simulink model "CAN_Model"  (R2018a)
settings: Solver=VariableStepAuto  StartTime=0.0  StopTime=12.4  RelTol=1e-3
InitFcn:
  | clc;
  | clear;
  | 
  | readyToSend = 1;
libraries: simulink_extras x2
settings Model: Creator=Emiliano  LastModifiedBy=Emiliano

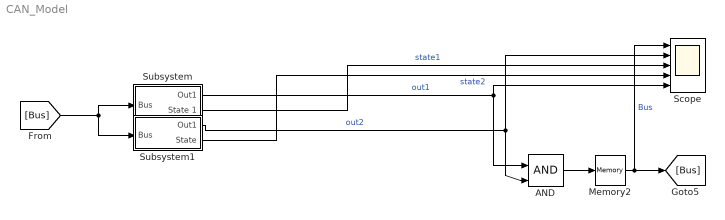
== system CAN_Model ==
  AND : Logic  IconShape=distinctive  AllPortsSameDT=off  OutDataTypeStr=boolean
  Memory2 : Memory  InitialCondition=1  InheritSampleTime=on
  Scope : Scope  NumInputPorts=5
  Subsystem : Subsystem
  Subsystem1 : Subsystem
  wires:
  AND/1 -> Memory2/1
  Memory2/1 -> Scope/1, [Bus]  "Bus"
  Subsystem/1(Out1) -> Scope/5, AND/1  "out1"
  Subsystem1/1(Out1) -> AND/2, Scope/2  "out2"
  [Bus] -> Subsystem1/1("Bus "), Subsystem/1("Bus ")
  Subsystem/2(State 1) -> Scope/3  "state1"
  Subsystem1/2("State ") -> Scope/4  "state2"

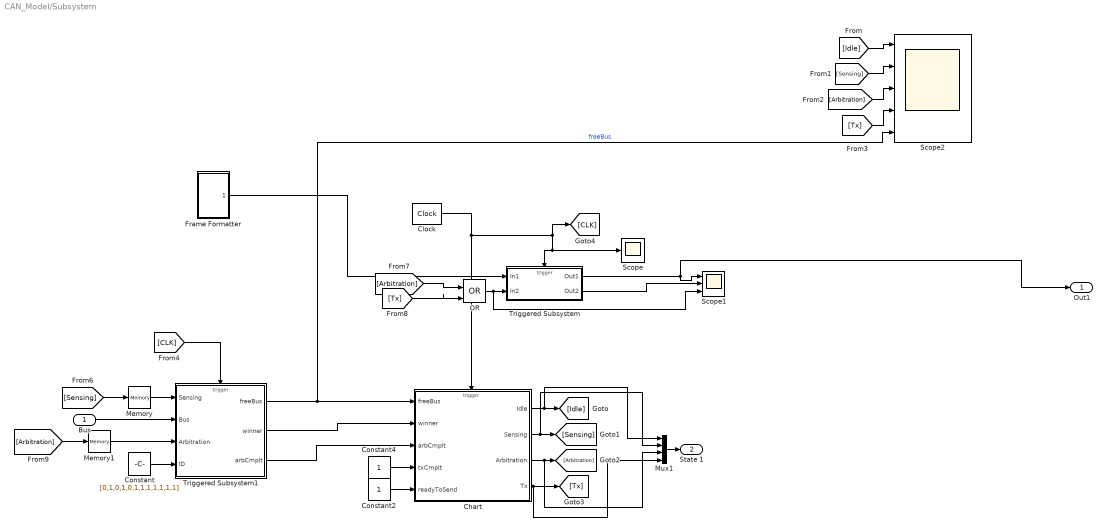
== system CAN_Model/Subsystem ==
  "Bus " : Inport
  Chart : Stateflow chart  TreatAsAtomicUnit=on
  Clock : simulink_extras/Flip Flops/Clock  period=0.2
  Constant : Constant  Value=[0,1,0,1,0,1,1,1,1,1,1,1]
  Constant2 : Constant
  Constant4 : Constant
  Frame Formatter : Subsystem
  Memory : Memory  InheritSampleTime=on
  Memory1 : Memory
  Mux1 : Mux
  OR : Logic  Operator=OR  IconShape=distinctive  AllPortsSameDT=off  OutDataTypeStr=boolean
  Scope : Scope
  Scope1 : Scope  NumInputPorts=3
  Scope2 : Scope  NumInputPorts=5
  Triggered Subsystem : Subsystem  TreatAsAtomicUnit=on
  Triggered Subsystem1 : Subsystem  TreatAsAtomicUnit=on
  Out1 : Outport
  State 1 : Outport  Port=2
  wires:
  Constant/1 -> Triggered Subsystem1/4(ID)
  Clock/1 -> Chart/Trigger, [CLK], Triggered Subsystem/Trigger, Scope/1
  OR/1 -> Scope1/3, Triggered Subsystem/2(In2)
  [Arbitration] -> OR/1
  Memory1/1 -> Triggered Subsystem1/3("Arbitration ")
  Triggered Subsystem1/3(arbCmplt) -> Chart/3(arbCmplt)
  Triggered Subsystem1/2(winner) -> Chart/2(winner)
  [Idle] -> Scope2/1
  [Tx] -> OR/2
  Constant2/1 -> Chart/5(readyToSend)
  [Arbitration] -> Memory1/1
  Memory/1 -> Triggered Subsystem1/1(Sensing)
  Triggered Subsystem1/1("freeBus ") -> Chart/1(freeBus), Scope2/5  "freeBus"
  [CLK] -> Triggered Subsystem1/Trigger
  [Sensing] -> Memory/1
  Frame Formatter/1(Frame) -> Triggered Subsystem/1(In1)
  Constant4/1 -> Chart/4(txCmplt)
  Triggered Subsystem/2(Out2) -> Scope1/2
  Triggered Subsystem/1(Out1) -> Out1/1, Scope1/1
  [Tx] -> Scope2/4
  [Arbitration] -> Scope2/3
  [Sensing] -> Scope2/2
  "Bus "/1 -> Triggered Subsystem1/2(Bus)
  Chart/2(" Sensing") -> [Sensing], Mux1/2
  Chart/4(" Tx") -> Mux1/4, [Tx]
  Chart/1(" Idle") -> [Idle], Mux1/1
  Chart/3(" Arbitration") -> Mux1/3, [Arbitration]
  Mux1/1 -> State 1/1

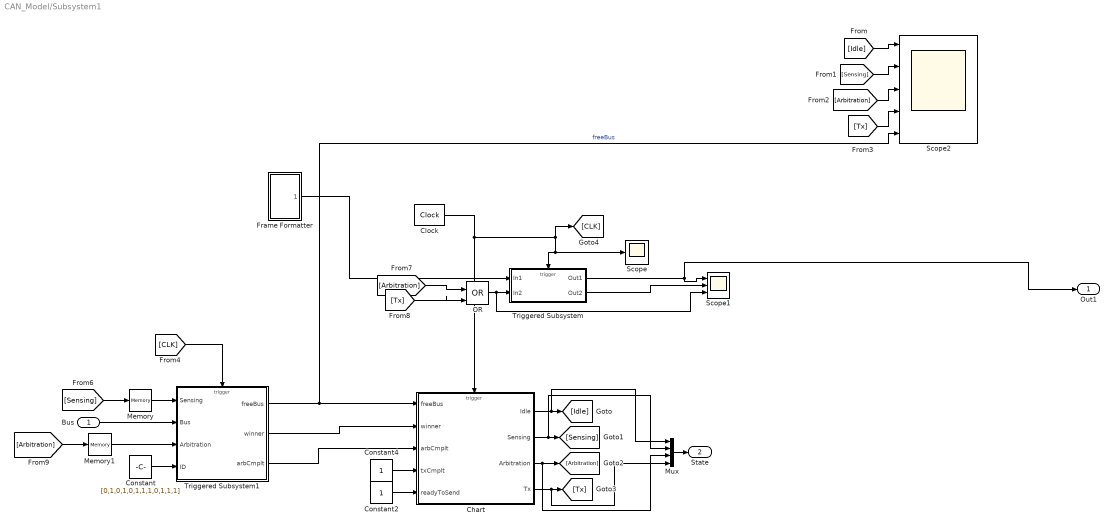
== system CAN_Model/Subsystem1 ==
  "Bus " : Inport
  Chart : Stateflow chart  TreatAsAtomicUnit=on
  Clock : simulink_extras/Flip Flops/Clock  period=0.2
  Constant : Constant  Value=[0,1,0,1,0,1,1,1,0,1,1,1]
  Constant2 : Constant
  Constant4 : Constant
  Frame Formatter : Subsystem
  Memory : Memory  InheritSampleTime=on
  Memory1 : Memory
  Mux : Mux
  OR : Logic  Operator=OR  IconShape=distinctive  AllPortsSameDT=off  OutDataTypeStr=boolean
  Scope : Scope
  Scope1 : Scope  NumInputPorts=3
  Scope2 : Scope  NumInputPorts=5
  Triggered Subsystem : Subsystem  TreatAsAtomicUnit=on
  Triggered Subsystem1 : Subsystem  TreatAsAtomicUnit=on
  Out1 : Outport
  "State " : Outport  Port=2
  wires:
  Constant/1 -> Triggered Subsystem1/4(ID)
  Clock/1 -> Chart/Trigger, [CLK], Triggered Subsystem/Trigger, Scope/1
  OR/1 -> Scope1/3, Triggered Subsystem/2(In2)
  [Arbitration] -> OR/1
  Memory1/1 -> Triggered Subsystem1/3("Arbitration ")
  Triggered Subsystem1/3(arbCmplt) -> Chart/3(arbCmplt)
  Triggered Subsystem1/2(winner) -> Chart/2(winner)
  [Idle] -> Scope2/1
  [Tx] -> OR/2
  Constant2/1 -> Chart/5(readyToSend)
  [Arbitration] -> Memory1/1
  Memory/1 -> Triggered Subsystem1/1(Sensing)
  Chart/4(" Tx") -> Mux/4, [Tx]
  Triggered Subsystem1/1("freeBus ") -> Chart/1(freeBus), Scope2/5  "freeBus"
  Chart/2(" Sensing") -> Mux/2, [Sensing]
  [CLK] -> Triggered Subsystem1/Trigger
  Chart/1(" Idle") -> Mux/1, [Idle]
  Chart/3(" Arbitration") -> Mux/3, [Arbitration]
  [Sensing] -> Memory/1
  Frame Formatter/1(Frame) -> Triggered Subsystem/1(In1)
  Constant4/1 -> Chart/4(txCmplt)
  Triggered Subsystem/2(Out2) -> Scope1/2
  Triggered Subsystem/1(Out1) -> Out1/1, Scope1/1
  [Tx] -> Scope2/4
  [Arbitration] -> Scope2/3
  [Sensing] -> Scope2/2
  "Bus "/1 -> Triggered Subsystem1/2(Bus)
  Mux/1 -> "State "/1

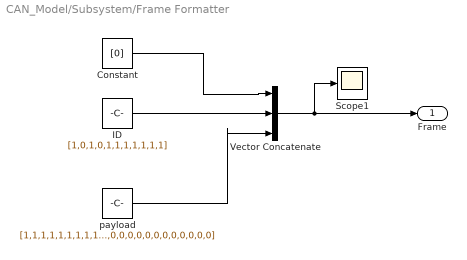
== system CAN_Model/Subsystem/Frame Formatter ==
  Constant : Constant  Value=[0]
  ID : Constant  Value=[1,0,1,0,1,1,1,1,1,1,1]
  Scope1 : Scope
  Vector Concatenate : Concatenate  NumInputs=3
  "payload " : Constant  Value=[1,1,1,1,1,1,1,1,1,1,1,1,1,1,1,1,1,1,1,1,1,1,1,1,1,0,0,0,0,0,0,0,0,0,0,0,0,0,0,0,0,0,0,0,0,0,0,0,0,0]
  Frame : Outport
  wires:
  ID/1 -> Vector Concatenate/2
  Constant/1 -> Vector Concatenate/1
  "payload "/1 -> Vector Concatenate/3
  Vector Concatenate/1 -> Frame/1, Scope1/1

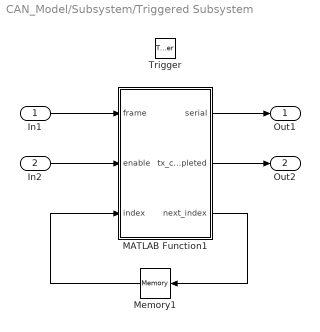
== system CAN_Model/Subsystem/Triggered Subsystem ==
  In1 : Inport
  In2 : Inport  Port=2
  Trigger : TriggerPort  VariantControl=Variant
  MATLAB Function1 : MATLAB Function  TreatAsAtomicUnit=on
  Memory1 : Memory  InitialCondition=1  InheritSampleTime=on
  Out1 : Outport
  Out2 : Outport  Port=2
  wires:
  In1/1 -> MATLAB Function1/1(frame)
  Memory1/1 -> MATLAB Function1/3(index)
  MATLAB Function1/1(serial) -> Out1/1
  MATLAB Function1/3(next_index) -> Memory1/1
  MATLAB Function1/2(tx_completed) -> Out2/1
  In2/1 -> MATLAB Function1/2(enable)

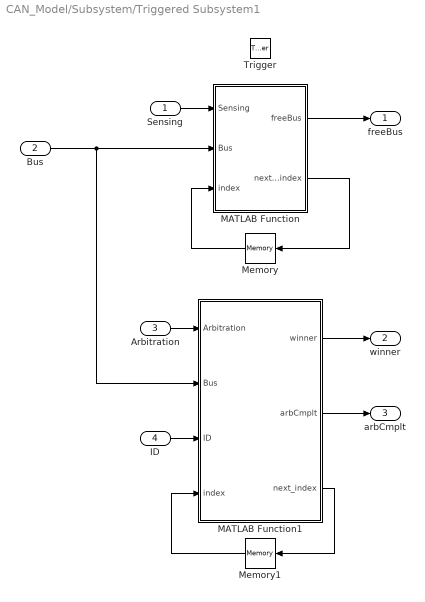
== system CAN_Model/Subsystem/Triggered Subsystem1 ==
  Sensing : Inport
  Bus : Inport  Port=2
  "Arbitration " : Inport  Port=3
  ID : Inport  Port=4
  Trigger : TriggerPort  VariantControl=Variant
  MATLAB Function : MATLAB Function  TreatAsAtomicUnit=on
  MATLAB Function1 : MATLAB Function  TreatAsAtomicUnit=on
  Memory : Memory  InheritSampleTime=on
  Memory1 : Memory  InitialCondition=1  InheritSampleTime=on
  "freeBus " : Outport
  winner : Outport  Port=2
  arbCmplt : Outport  Port=3
  wires:
  Sensing/1 -> MATLAB Function/1(Sensing)
  Bus/1 -> MATLAB Function1/2(Bus), MATLAB Function/2(Bus)
  MATLAB Function/2(next_index) -> Memory/1
  Memory/1 -> MATLAB Function/3(index)
  MATLAB Function/1(freeBus) -> "freeBus "/1
  "Arbitration "/1 -> MATLAB Function1/1(Arbitration)
  MATLAB Function1/3(next_index) -> Memory1/1
  Memory1/1 -> MATLAB Function1/4(index)
  ID/1 -> MATLAB Function1/3(ID)
  MATLAB Function1/2(arbCmplt) -> arbCmplt/1
  MATLAB Function1/1(winner) -> winner/1

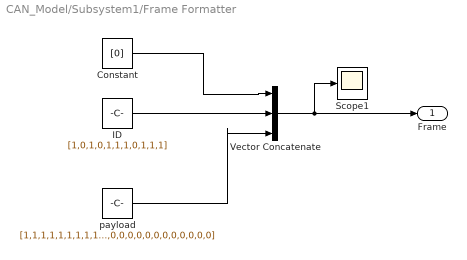
== system CAN_Model/Subsystem1/Frame Formatter ==
  Constant : Constant  Value=[0]
  ID : Constant  Value=[1,0,1,0,1,1,1,0,1,1,1]
  Scope1 : Scope
  Vector Concatenate : Concatenate  NumInputs=3
  "payload " : Constant  Value=[1,1,1,1,1,1,1,1,1,1,1,1,1,1,1,1,1,1,1,1,1,1,1,1,1,0,0,0,0,0,0,0,0,0,0,0,0,0,0,0,0,0,0,0,0,0,0,0,0,0]
  Frame : Outport
  wires:
  ID/1 -> Vector Concatenate/2
  Constant/1 -> Vector Concatenate/1
  "payload "/1 -> Vector Concatenate/3
  Vector Concatenate/1 -> Frame/1, Scope1/1

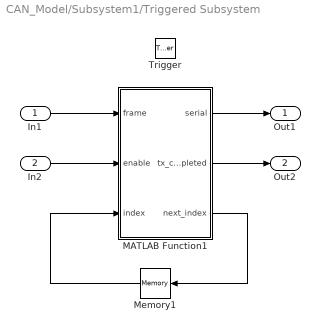
== system CAN_Model/Subsystem1/Triggered Subsystem ==
  In1 : Inport
  In2 : Inport  Port=2
  Trigger : TriggerPort  VariantControl=Variant
  MATLAB Function1 : MATLAB Function  TreatAsAtomicUnit=on
  Memory1 : Memory  InitialCondition=1  InheritSampleTime=on
  Out1 : Outport
  Out2 : Outport  Port=2
  wires:
  In1/1 -> MATLAB Function1/1(frame)
  Memory1/1 -> MATLAB Function1/3(index)
  MATLAB Function1/1(serial) -> Out1/1
  MATLAB Function1/3(next_index) -> Memory1/1
  MATLAB Function1/2(tx_completed) -> Out2/1
  In2/1 -> MATLAB Function1/2(enable)

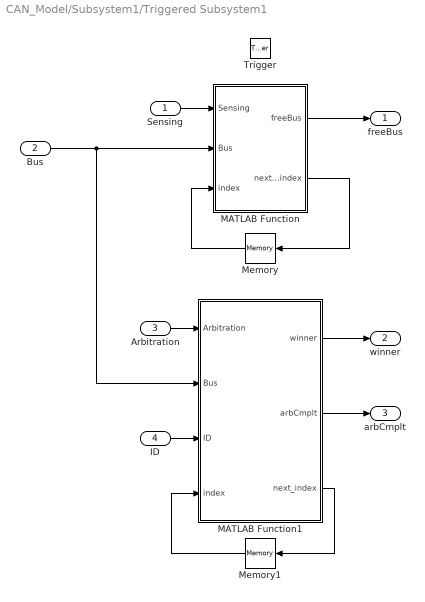
== system CAN_Model/Subsystem1/Triggered Subsystem1 ==
  Sensing : Inport
  Bus : Inport  Port=2
  "Arbitration " : Inport  Port=3
  ID : Inport  Port=4
  Trigger : TriggerPort  VariantControl=Variant
  MATLAB Function : MATLAB Function  TreatAsAtomicUnit=on
  MATLAB Function1 : MATLAB Function  TreatAsAtomicUnit=on
  Memory : Memory  InheritSampleTime=on
  Memory1 : Memory  InitialCondition=1  InheritSampleTime=on
  "freeBus " : Outport
  winner : Outport  Port=2
  arbCmplt : Outport  Port=3
  wires:
  Sensing/1 -> MATLAB Function/1(Sensing)
  Bus/1 -> MATLAB Function1/2(Bus), MATLAB Function/2(Bus)
  MATLAB Function/2(next_index) -> Memory/1
  Memory/1 -> MATLAB Function/3(index)
  MATLAB Function/1(freeBus) -> "freeBus "/1
  "Arbitration "/1 -> MATLAB Function1/1(Arbitration)
  MATLAB Function1/3(next_index) -> Memory1/1
  Memory1/1 -> MATLAB Function1/4(index)
  ID/1 -> MATLAB Function1/3(ID)
  MATLAB Function1/2(arbCmplt) -> arbCmplt/1
  MATLAB Function1/1(winner) -> winner/1

== matlab function CAN_Model/Subsystem/Triggered Subsystem1/MATLAB Function ==
  data: Sensing input; freeBus output; Bus input; index input; next_index output
function [freeBus, next_index] = fcn(Sensing, Bus, index)

freeBus = 0;

if Sensing == 1
    if Bus == 1
        if index < 10
            next_index = index + 1;
        else
            next_index = 0;
            freeBus = 1;
        end
    else
        next_index = 0;
    end
else
   next_index = 0;
end

end

== matlab function CAN_Model/Subsystem/Triggered Subsystem/MATLAB Function1 ==
  data: frame input; enable input; serial output; tx_completed output; index input; next_index output
function [serial,  tx_completed ,next_index]  = fcn(frame, enable, index)

if enable == 1
frame_size = size(frame);
if index > frame_size
    serial = 1;
    tx_completed = 1;
    next_index = 1;
else
    serial = frame(index);
    next_index = index + 1;
    tx_completed = 0;
end
else
    tx_completed = 0;
    serial = 1;
    next_index = 1;
end

end

== stateflow chart CAN_Model/Subsystem/Chart ==
  settings: executeAtInitialization=1
  state Idle
  state Sensing
  state Tx
  state Arbitration
  (default) -> Idle
  Idle -> Idle [order 2] : [readyToSend == 0]
  Idle -> Sensing [order 1] : [readyToSend > 0]
  Tx -> Idle [order 1] : [txCmplt == 1]
  Sensing -> Sensing [order 1] : [freeBus == 0]
  Arbitration -> Sensing [order 2] : [winner == 0 && arbCmplt == 1]
  Tx -> Tx [order 2] : [txCmplt == 0]
  Sensing -> Arbitration [order 2] : [freeBus == 1]
  Arbitration -> Tx [order 1] : [winner == 1 && arbCmplt == 1]
  Arbitration -> Arbitration [order 3] : [arbCmplt == 0]
  data: freeBus input; winner input; Idle output boolean; Sensing output boolean; Arbitration output boolean; Tx output boolean; arbCmplt input; txCmplt input; readyToSend input
  events: Start input RISING_EDGE_EVENT

== matlab function CAN_Model/Subsystem/Triggered Subsystem1/MATLAB Function1 ==
  data: winner output; arbCmplt output; Arbitration input; Bus input; ID input; next_index output; index input
function [winner, arbCmplt, next_index] = fcn(Arbitration, Bus, ID, index)

arbCmplt = 0;
winner = 0;
next_index = 1;

if Arbitration == 1
    if index <= 12 
        if ID(index) == Bus
            next_index = index + 1;
        else
            winner = 0;
            arbCmplt = 1;
        end
    else
        next_index = 1;
        winner = 1;
        arbCmplt = 1;
    end    
    
else next_index = 1;
    
end
end

== stateflow chart CAN_Model/Subsystem1/Chart ==
  settings: executeAtInitialization=1
  state Idle
  state Sensing
  state Tx
  state Arbitration
  (default) -> Idle
  Idle -> Idle [order 2] : [readyToSend == 0]
  Idle -> Sensing [order 1] : [readyToSend > 0]
  Tx -> Idle [order 1] : [txCmplt == 1]
  Sensing -> Sensing [order 1] : [freeBus == 0]
  Arbitration -> Sensing [order 2] : [winner == 0 && arbCmplt == 1]
  Tx -> Tx [order 2] : [txCmplt == 0]
  Sensing -> Arbitration [order 2] : [freeBus == 1]
  Arbitration -> Tx [order 1] : [winner == 1 && arbCmplt == 1]
  Arbitration -> Arbitration [order 3] : [arbCmplt == 0]
  data: freeBus input; winner input; Idle output boolean; Sensing output boolean; Arbitration output boolean; Tx output boolean; arbCmplt input; txCmplt input; readyToSend input
  events: Start input RISING_EDGE_EVENT

== matlab function CAN_Model/Subsystem1/Triggered Subsystem/MATLAB Function1 ==
  data: frame input; enable input; serial output; tx_completed output; index input; next_index output
function [serial,  tx_completed ,next_index]  = fcn(frame, enable, index)

if enable == 1
frame_size = size(frame);
if index > frame_size
    serial = 1;
    tx_completed = 1;
    next_index = 1;
else
    serial = frame(index);
    next_index = index + 1;
    tx_completed = 0;
end
else
    tx_completed = 0;
    serial = 1;
    next_index = 1;
end

end

== matlab function CAN_Model/Subsystem1/Triggered Subsystem1/MATLAB Function ==
  data: Sensing input; freeBus output; Bus input; index input; next_index output
function [freeBus, next_index] = fcn(Sensing, Bus, index)

freeBus = 0;

if Sensing == 1
    if Bus == 1
        if index < 10
            next_index = index + 1;
        else
            next_index = 0;
            freeBus = 1;
        end
    else
        next_index = 0;
    end
else
   next_index = 0;
end

end

== matlab function CAN_Model/Subsystem1/Triggered Subsystem1/MATLAB Function1 ==
  data: winner output; arbCmplt output; Arbitration input; Bus input; ID input; next_index output; index input
function [winner, arbCmplt, next_index] = fcn(Arbitration, Bus, ID, index)

arbCmplt = 0;
winner = 0;
next_index = 1;

if Arbitration == 1
    if index <= 12 
        if ID(index) == Bus
            next_index = index + 1;
        else
            winner = 0;
            arbCmplt = 1;
        end
    else
        next_index = 1;
        winner = 1;
        arbCmplt = 1;
    end    
    
else next_index = 1;
    
end
end
